simulink model "wing_beat_model"  (R2021a)
settings: Solver=VariableStepAuto  StartTime=0.0  StopTime=10.0  RelTol=1e-3
settings Model: Creator=Nabil  LastModifiedBy=Nabil

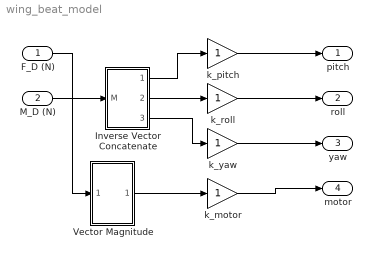
== system wing_beat_model ==
  F_D (N) : Inport  PortDimensions=3
  M_D (N) : Inport  Port=2
  Inverse Vector Concatenate : Subsystem
  Vector Magnitude : Subsystem
  k_motor : Gain
  k_pitch : Gain
  k_roll : Gain
  k_yaw : Gain
  pitch : Outport
  roll : Outport  Port=2
  yaw : Outport  Port=3
  motor : Outport  Port=4
  wires:
  k_pitch/1 -> pitch/1
  k_roll/1 -> roll/1
  k_yaw/1 -> yaw/1
  k_motor/1 -> motor/1
  F_D (N)/1 -> Vector Magnitude/1(In1)
  Vector Magnitude/1(Out1) -> k_motor/1
  Inverse Vector Concatenate/1(Out1) -> k_pitch/1
  Inverse Vector Concatenate/2(Out2) -> k_roll/1
  Inverse Vector Concatenate/3(Out3) -> k_yaw/1
  M_D (N)/1 -> Inverse Vector Concatenate/1(M)

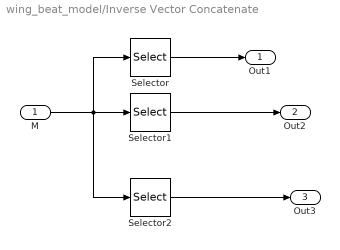
== system wing_beat_model/Inverse Vector Concatenate ==
  M : Inport
  Selector : Selector  InputPortWidth=3  IndexOptions=Index vector (dialog)  Indices=1  OutputSizes=1
  Selector1 : Selector  InputPortWidth=3  IndexOptions=Index vector (dialog)  Indices=2  OutputSizes=1
  Selector2 : Selector  InputPortWidth=3  IndexOptions=Index vector (dialog)  Indices=3  OutputSizes=1
  Out1 : Outport
  Out2 : Outport  Port=2
  Out3 : Outport  Port=3
  wires:
  Selector1/1 -> Out2/1
  M/1 -> Selector2/1, Selector/1, Selector1/1
  Selector2/1 -> Out3/1
  Selector/1 -> Out1/1

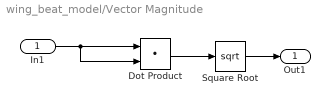
== system wing_beat_model/Vector Magnitude ==
  In1 : Inport
  Dot Product : DotProduct  InputSameDT=on  OutDataTypeStr=Inherit: Inherit via internal rule
  Square Root : Sqrt  SaturateOnIntegerOverflow=on
  Out1 : Outport
  wires:
  In1/1 -> Dot Product/2, Dot Product/1
  Dot Product/1 -> Square Root/1
  Square Root/1 -> Out1/1
